simulink model "soc_top"  (R2023b)
settings: Solver=VariableStepAuto  StartTime=0.0  StopTime=0.5  FixedStep=1e-09  RelTol=1e-3  EnableMultiTasking=on
model workspace (MAT data in the model file):
  socvcb = containers.Map
  socvcb.serialization.keys = {25710.0247803, 26285.0009766, 32862.0010986}
  socvcb.serialization.values : function handle (value not decoded)
  socvcb.serialization.uniformity = 0
  socvcb.serialization.keyType = 'double'
  socvcb.serialization.valueType = 'any'
libraries: socmemlib x2, proctasklib x1
settings Model: Creator=user poco smart  LastModifiedBy=user poco smart
settings SolverCC: ConcurrentTasks=on  AlgebraicLoopSolver=TrustRegion  PositivePriorityOrder=on  AutoInsertRateTranBlk=on  MinimalZcImpactIntegration=on  MaxZcPerStep=1
settings DataIOCC: ReturnWorkspaceOutputs=off
settings OptimizationCC: EnhancedBackFolding=on  PassReuseOutputArgsAs=Individual arguments  MaxStackSize=64  OptimizeBlockOrder=speed  DifferentSizesBufferReuse=on  OptimizationCustomize=off  EfficientTunableParamExpr=on
settings DebuggingCC: IntegerOverflowMsg=none  ParameterPrecisionLossMsg=none  ParameterTunabilityLossMsg=error  UnconnectedInputMsg=warning  UnconnectedOutputMsg=warning  UnconnectedLineMsg=warning  PregeneratedLibrarySubsystemCodeDiagnostic=none  ArithmeticOperatorsInVariantConditions=warning
settings HardwareCC: ProdBitPerPointer=32  ProdBitPerSizeT=32  ProdBitPerPtrDiffT=32  ProdLargestAtomicInteger=Long  ProdLargestAtomicFloat=Double  ProdWordSize=32  ProdLongLongMode=on  ProdHWDeviceType=ARM Compatible->ARM Cortex-A (32-bit)  HardwareBoardFeatureSet=SoCBlockset
settings ModelReferenceCC: ModelReferenceNumInstancesAllowed=Single
settings SFSimCC: SimUseLocalCustomCode=off  MATLABDynamicMemAlloc=off  CustomCodeUndefinedFunction=UseInterfaceOnly
settings RTWCC: Description=Embedded Coder  SystemTargetFile=ert.tlc  HardwareBoard=ZedBoard  TLCOptions="-aInlineSetEventsForThisBaseRateFcn=TLC_FALSE -aSuppressMultiTaskScheduler=TLC_FALSE  -aRateBasedStepFcn=0"  TemplateMakefile=ert_default_tmf  GenerateReport=on  RTWUseLocalCustomCode=off  Toolchain=Linaro AArch32 Linux v6.3.1  IncludeHyperlinkInReport=on  LaunchReport=on  GenerateTraceInfo=on  GenerateTraceReport=on  GenerateTraceReportSl=on  GenerateTraceReportSf=on  GenerateTraceReportEml=on  DLArmComputeVersion=19.05
settings CodeAppCC: ForceParamTrailComments=on  IgnoreCustomStorageClasses=off  OperatorAnnotations=on  SimulinkDataObjDesc=on  SFDataObjDesc=on  InsertBlockDesc=on
settings ERTTargetCC: ExtModeTransport=2  ExtModeStaticAlloc=on  ExtModeMexFile=ext_xcp  ExtModeIntrfLevel=Level2 - Open
settings ConfigComp: CovBoundaryAbsTol=1.0e-5
settings SettingsController: UseSoCProfilerForTargets=0

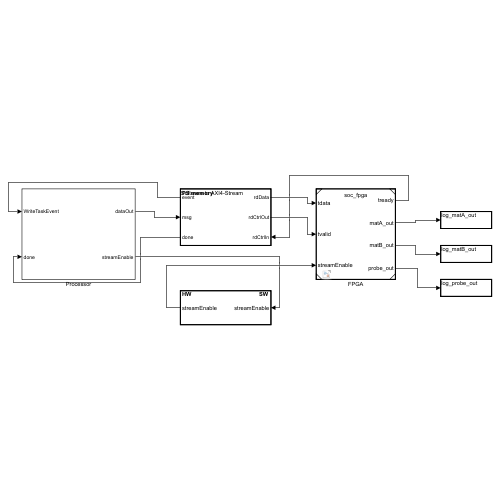
[thumbnail: Simulink's stored preview of the top-level diagram]
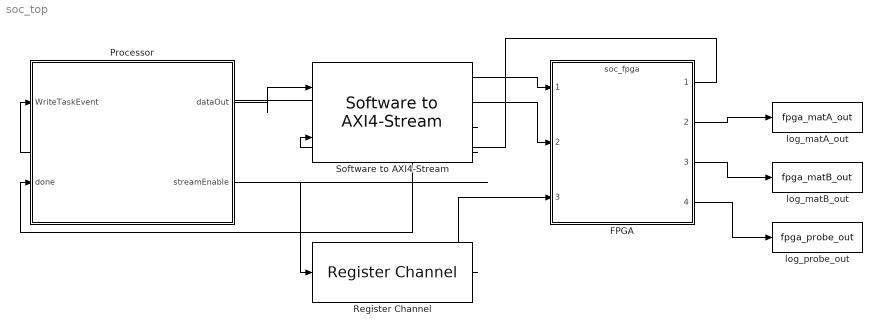
== system soc_top ==
  FPGA : ModelReference  ModelNameDialog=soc_fpga.slx  SimulationMode=Normal  ModelReferenceVersion=1.0
  Processor : Subsystem
  Register Channel : socmemlib/Register Channel  RegisterTable={'streamEnable','Write','boolean','1','0'}  SampleTime=-1  RegTableNames={'streamEnable'}  RegTableRW={'Write'}  RegTableDataTypes={'boolean'}  RegTableVectorSizes={'1'}  NumRegisters=1  RegTableInitialValues={'0' }  RegTableDirty=1
  Software to AXI4-Stream : socmemlib/Software to AXI4-Stream  MemorySimulation=Burst accurate  MemorySelection=PS memory  MRNumBuffers=8  BurstLengthReaderChIf=25  FIFODepthReader=8  FIFOAFullDepthReader=6  ICClockFrequencyReader=100  ICDataWidthReader=32  ChDimensionsWriterChIf=25  ChTypeWriterChIf=uint32  ChDimensionsReaderChIf=25  ChTypeReaderChIf=int32  ChFrameSampleTimeReaderChIf=0.10000000000000001  ChBitPackedReaderChIf=off  EnableMemSim=on  LastTargetBoard=ZedBoard  MRRegionSize=800  MRBufferSize=100  DiagnosticLevel=No debug  ChFrameSampleTimeWriterChIf=[0.1 0]  ChBitPackedWriterChIf=off  BurstLengthWriterChIf=256  FIFODepthWriter=8  FIFOAFullDepthWriter=6  ICClockFrequencyWriter=100  ICDataWidthWriter=64
  log_matA_out : ToWorkspace  VariableName=fpga_matA_out  SaveFormat=Timeseries  SampleTime=-1
  log_matB_out : ToWorkspace  VariableName=fpga_matB_out  SaveFormat=Timeseries  SampleTime=-1
  log_probe_out : ToWorkspace  VariableName=fpga_probe_out  SaveFormat=Timeseries  SampleTime=-1
  wires:
  Processor/1(dataOut) -> Software to AXI4-Stream/1
  FPGA/1 -> Software to AXI4-Stream/2
  Software to AXI4-Stream/1 -> FPGA/1
  Software to AXI4-Stream/2 -> FPGA/2
  Software to AXI4-Stream/3 -> Processor/1(WriteTaskEvent)
  Software to AXI4-Stream/4 -> Processor/2(done)
  Processor/2(streamEnable) -> Register Channel/1
  Register Channel/1 -> FPGA/3
  FPGA/2 -> log_matA_out/1
  FPGA/3 -> log_matB_out/1
  FPGA/4 -> log_probe_out/1

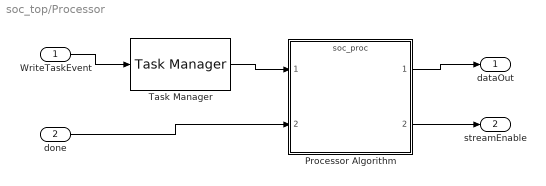
== system soc_top/Processor ==
  WriteTaskEvent : Inport
  done : Inport  Port=2
  Processor Algorithm : ModelReference  ModelNameDialog=soc_proc.slx  SimulationMode=Normal  ModelReferenceVersion=1.0
  Task Manager : proctasklib/Task Manager  AllTaskData="{\"taskName\":\"ComputeTask\",\"taskType\":\"Event-driven\",\"taskEvent\":\"ComputeTaskEvent\",\"taskPeriod\":\"0.1\",\"taskPriority\":\"50\",\"coreSelection\":\"Specified core\",\"coreNum\":\"0\",\"dropOverranTasks\":false,\"playbackRecorded\":false,\"diagnosticsFile\":\"\",\"taskDurationSource\":\"Dialog\",\"taskDuration\":1E-6,\"taskDurationDeviation\":0,\"logExecutionData\":true,\"logDroppedTasks\":false,\"version\":\"2.6\",\"taskDurationData\":{\"percent\":\"100\",\"mean\":\"1e-06\",\"dev\":\"0\",\"min\":\"1e-06\",\"max\":\"1e-06\"},\"taskEventSource\":\"Unspecified\",\"taskEventSourceAssignmentType\":\"Unassigned\",\"taskEventSourceType\":\"Unspecified\",\"taskEventGroup\":\"Unspecified\",\"taskEventInterrupt\":\"Unspecified\",\"taskEventOrder\":1,\"taskDisablePremption\":false,\"taskClearInterruptFlagsAtEndOfEvent\":false}"  EnableTaskSimulation=on  StreamToSDI=on  WriteToFile=off  OverwriteFile=off  SupportEventPorts=on  UseScheduleEditor=off  CustomizationInfo=''
  dataOut : Outport
  streamEnable : Outport  Port=2
  wires:
  WriteTaskEvent/1 -> Task Manager/1
  Task Manager/1 -> Processor Algorithm/1
  done/1 -> Processor Algorithm/2
  Processor Algorithm/1 -> dataOut/1
  Processor Algorithm/2 -> streamEnable/1
